simulink model "EngineTorqueController"  (R2015a)
settings: Solver=ode3  SolverMode=SingleTasking  StartTime=0.0  StopTime=inf  RelTol=1e-3
PreLoadFcn:
  | clear all
  | Kp =0.0614; Ki = 0.0723;
undefined symbols (not defined in the file): serial
libraries: instrumentlib x2
Description:
  | Engine Timing Model With Closed Loop Control
  | 
  | This demonstration shows how to use triggered subsystems in Simulink(R) to model
  | engine timing, including a feedback controller. Different subsystems in the diagram
  | model the mathematical representation of various automotive systems, including
  | the following:
  | 
  | * Throttle and manifold
  | * Compression
  | * Combustion
  | * Vehicle dynamics
  | * Valve timing
  | * Controller
  | 
  | The valve timing subsystem generates a signal that triggers the Controller and
  | Compression subsystems twice per revolution of the crank (calculated from the
  | crank speed.) A speed set point (in rpm) from the Step block drives the simulation.
  | The controller calculates the necessary throttle angle based on the desired rpm
  | and the crank speed that is calculated by the vehicle dynamics. After you run
  | the simulation, the Scopes show the engine speed and the throttle angle
  | compared to the load torque.
settings Model: CovMetricSettings=d  ExtModeTrigMode=oneshot  ExtModeTrigDuration=2  ExtModeArmWhenConnect=off  ExtModeAutoUpdateStatusClock=off  Creator=The MathWorks Inc.  LastModifiedBy=Piyush
settings OptimizationCC: OptimizeModelRefInitCode=on  LifeSpan=1
settings DebuggingCC: UnderspecifiedInitializationDetection=Classic  MergeDetectMultiDrivingBlocksExec=none
settings HardwareCC: ProdBitPerInt=16  ProdBitPerPointer=8  ProdIntDivRoundTo=Zero  ProdEndianess=LittleEndian  ProdWordSize=8  ProdHWDeviceType=Atmel->AVR
settings RTWCC: SystemTargetFile=realtime.tlc  GenerateMakefile=off  TemplateMakefile=realtime.tmf  Description=Run on Target Hardware  RTWVerbose=off
settings ERTTargetCC: CombineOutputUpdateFcns=off  ExtModeTransport=3  ExtModeMexFile=ext_serial_win32_comm_rtt  ExtModeMexArgs=0 1 9600  ERTSrcFileBannerTemplate=realtime_code_template.cgt  ERTHdrFileBannerTemplate=realtime_code_template.cgt  ERTDataSrcFileTemplate=realtime_code_template.cgt  ERTDataHdrFileTemplate=realtime_code_template.cgt  ERTCustomFileTemplate=realtime_file_process.tlc

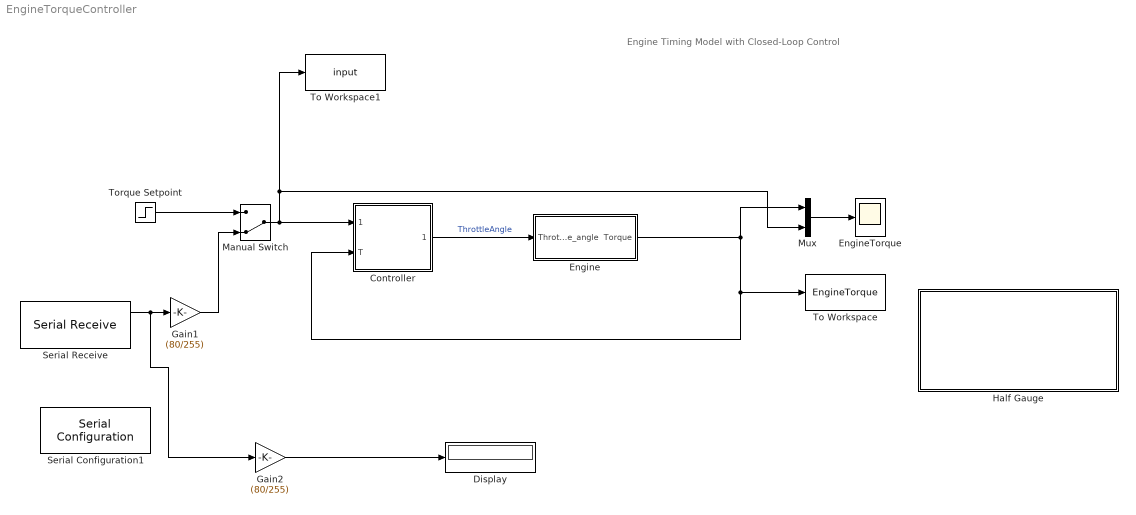
== system EngineTorqueController ==
  note: Engine Timing Model with Closed-Loop Control
  Controller : Subsystem  TreatAsAtomicUnit=on
  Display : Display
  Engine : Subsystem
  EngineTorque : Scope
      settings: TickLabels=on  TimeRange=10  YMin=39.9355  YMax=39.9355  SaveName=EngineSpeed  DataFormat=Structure
  Gain1 : Gain  Gain=(80/255)
  Gain2 : Gain  Gain=(80/255)
  Half Gauge : Subsystem  DialogController=hmiCreateDDGDialog  IsWebBlock=on  mask(MathWorksWebBlock){webBlockId=42deb273-d939-4e08-ae5d-adf02b1defd7, webBlockType=semicirculargauge, ShowInLibBrowser=on, ShowInitialText=on, HMISrcModelName=Main_EngineTorqueController}
      mask prompts: webBlockId "WebBlock Id"; webBlockType "WebBlock Type"; HMISrcModelName "Source Model"
      mask Help: helpview([docroot '/mapfiles/simulink.map'], 'hmi_half_gauge')
      mask Display:
      | if strcmp(get_param(bdroot(gcb),'BlockDiagramType'), 'library')
      |     image([(matlabroot) '/toolbox/simulink/hmi/icons/SemicircularGauge.png']);
      | end
  Manual Switch : ManualSwitch  CurrentSetting=0
  Mux : Mux  Inputs=2
  Serial Configuration1 : instrumentlib/Serial Configuration  Priority=-200000  ComPortMenu=<Please select a port...>  ComPort=COM4  ObjConstructor=serial('COM4');  BaudRate=9600  DataBits=8  Parity=none  StopBits=1  FlowControl=none  Timeout=10  ByteOrder=BigEndian
  Serial Receive : instrumentlib/Serial Receive  ComPortMenu=<Please select a port...>  ComPort=COM4  ObjConstructor=serial('COM4');  Terminator=<none>  DataSize=[1 1]  DataType=uint8  EnableBlockingMode=off  ActionDataUnavailable=Output last received value  CustomValue=0  SampleTime=0.01
  To Workspace : ToWorkspace  VariableName=EngineTorque  SaveFormat=Timeseries  SampleTime=-1
  To Workspace1 : ToWorkspace  VariableName=input  SaveFormat=Timeseries  SampleTime=-1
  Torque Setpoint : Step  Time=5  Before=30  After=40  SampleTime=0
  wires:
  Manual Switch/1 -> Mux/2, To Workspace1/1, Controller/1(Desired Torque)
  Controller/1(Throttle Ang.) -> Engine/1(Throttle_angle)  "ThrottleAngle"
  Engine/1(Torque) -> Mux/1, Controller/2(T), To Workspace/1
  Mux/1 -> EngineTorque/1
  Torque Setpoint/1 -> Manual Switch/1
  Serial Receive/1 -> Gain2/1, Gain1/1
  Gain1/1 -> Manual Switch/2
  Gain2/1 -> Display/1

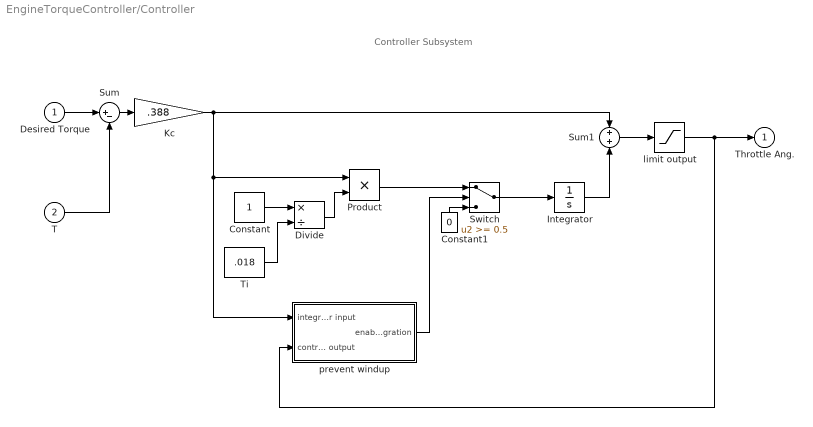
== system EngineTorqueController/Controller ==
  note: Controller Subsystem
  Desired Torque : Inport
  T : Inport  Port=2
  Constant : Constant
  Constant1 : Constant  Value=0
  Divide : Product  Inputs=*/
  Integrator : Integrator  ZeroCross=off
  Kc : Gain  Gain=.388  SaturateOnIntegerOverflow=on  OutDataTypeStr=Inherit: Same as input  ParamDataTypeStr=Inherit: Same as input
  Product : Product
  Sum : Sum  Inputs=|+-  SaturateOnIntegerOverflow=on  InputSameDT=on  OutDataTypeStr=Inherit: Same as first input
  Sum1 : Sum  SaturateOnIntegerOverflow=on  InputSameDT=on  OutDataTypeStr=Inherit: Same as first input
  Switch : Switch  Threshold=0.5  SaturateOnIntegerOverflow=on  InputSameDT=on
  Ti : Constant  Value=.018
  limit output : Saturate  UpperLimit=70  LowerLimit=0
  prevent windup : Subsystem
  Throttle Ang. : Outport  InitialOutput=8.973
  wires:
  Desired Torque/1 -> Sum/1
  Integrator/1 -> Sum1/2
  limit output/1 -> prevent windup/2(controller output), Throttle Ang./1
  prevent windup/1(enable integration) -> Switch/2
  Sum1/1 -> limit output/1
  Switch/1 -> Integrator/1
  Kc/1 -> Sum1/1, prevent windup/1(integrator input), Product/1
  Constant1/1 -> Switch/3
  Product/1 -> Switch/1
  Sum/1 -> Kc/1
  T/1 -> Sum/2
  Constant/1 -> Divide/1
  Ti/1 -> Divide/2
  Divide/1 -> Product/2

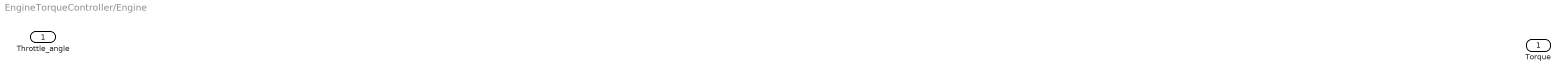
== system EngineTorqueController/Engine ==
  Throttle_angle : Inport
  Torque : Outport

== system EngineTorqueController/Half Gauge ==

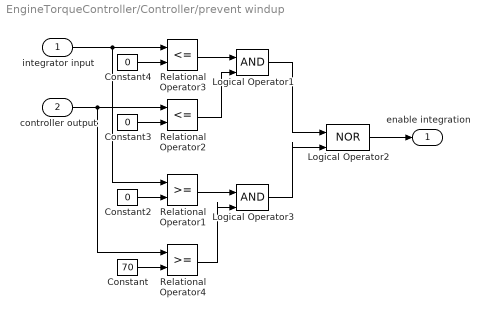
== system EngineTorqueController/Controller/prevent windup ==
  integrator input : Inport
  controller output : Inport  Port=2
  Constant : Constant  Value=70
  Constant2 : Constant  Value=0
  Constant3 : Constant  Value=0
  Constant4 : Constant  Value=0
  Logical Operator1 : Logic  IconShape=distinctive
  Logical Operator2 : Logic  Operator=NOR  IconShape=distinctive
  Logical Operator3 : Logic  IconShape=distinctive
  Relational Operator1 : RelationalOperator  InputSameDT=on
  Relational Operator2 : RelationalOperator  Operator=<=  InputSameDT=on
  Relational Operator3 : RelationalOperator  Operator=<=  InputSameDT=on
  Relational Operator4 : RelationalOperator  InputSameDT=on
  enable integration : Outport  InitialOutput=0
  wires:
  Logical Operator2/1 -> enable integration/1
  Logical Operator3/1 -> Logical Operator2/2
  Logical Operator1/1 -> Logical Operator2/1
  Relational Operator4/1 -> Logical Operator3/2
  Relational Operator1/1 -> Logical Operator3/1
  Constant/1 -> Relational Operator4/2
  Constant2/1 -> Relational Operator1/2
  controller output/1 -> Relational Operator4/1, Relational Operator2/1
  integrator input/1 -> Relational Operator3/1, Relational Operator1/1
  Relational Operator2/1 -> Logical Operator1/2
  Relational Operator3/1 -> Logical Operator1/1
  Constant4/1 -> Relational Operator3/2
  Constant3/1 -> Relational Operator2/2
